simulink model "Mass_Spring_simulink"  (R2015a)
settings: Solver=ode8  StartTime=0.0  StopTime=300  FixedStep=0.0001  RelTol=1e-3
values from neighbouring files (symbols this model uses):
  B = 30    [Practice_mass_spring_sys_bySimulink.m]
  f = 300    [Practice_mass_spring_sys_bySimulink.m]
  K = 15    [Practice_mass_spring_sys_bySimulink.m]
  M = 750    [Practice_mass_spring_sys_bySimulink.m]
settings Model: Creator=DELL  LastModifiedBy=DELL

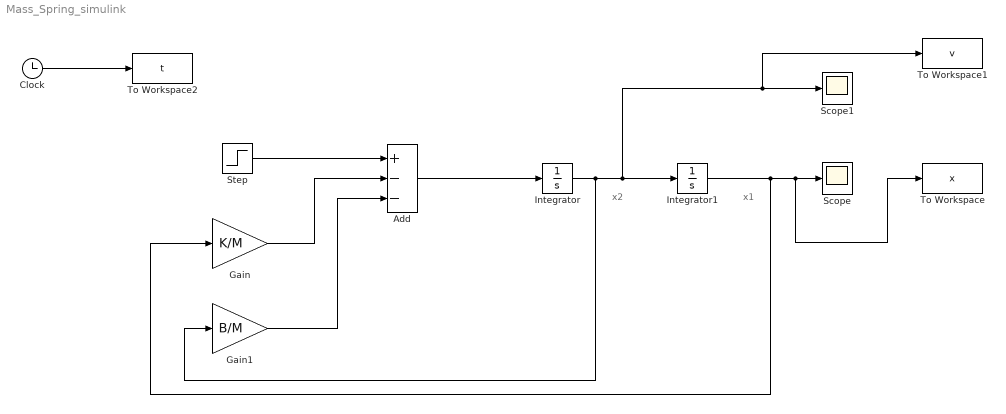
== system Mass_Spring_simulink ==
  note: x1
  note: x2
  Add : Sum  Inputs=+--
  Clock : Clock
  Gain : Gain  Gain=K/M
  Gain1 : Gain  Gain=B/M
  Integrator : Integrator
  Integrator1 : Integrator
  Scope : Scope
  Scope1 : Scope
  Step : Step  Time=0  After=f/M  SampleTime=0
  To Workspace : ToWorkspace  VariableName=x  SampleTime=-1
  To Workspace1 : ToWorkspace  VariableName=v  SampleTime=-1
  To Workspace2 : ToWorkspace  VariableName=t  SampleTime=-1
  wires:
  Integrator/1 -> Gain1/1, To Workspace1/1, Scope1/1, Integrator1/1
  Integrator1/1 -> Gain/1, To Workspace/1, Scope/1
  Add/1 -> Integrator/1
  Step/1 -> Add/1
  Gain/1 -> Add/2
  Gain1/1 -> Add/3
  Clock/1 -> To Workspace2/1
